simulink model "Clutch_control"  (R2020a)
settings: Solver=VariableStepAuto  StartTime=0.0  StopTime=10.0  RelTol=1e-3
undefined symbols (not defined in the file or in its folder): be, bv, Ie, Iv, lv, muk, mus, R
settings Model: Creator=DELL  LastModifiedBy=DELL

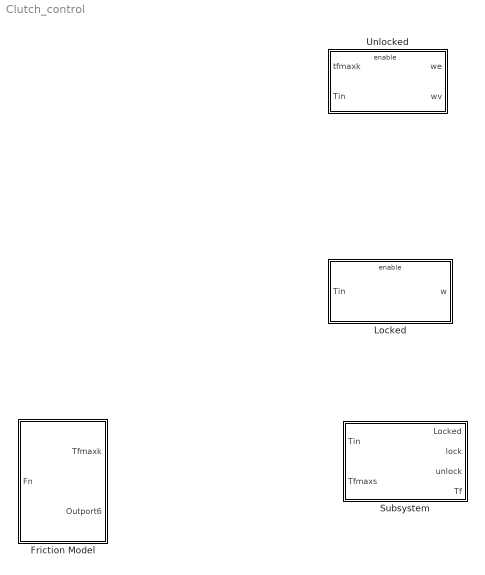
== system Clutch_control ==
  Friction Model : Subsystem
  Locked : Subsystem
  Subsystem : Subsystem
  Unlocked : Subsystem

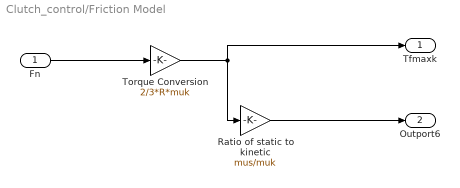
== system Clutch_control/Friction Model ==
  Fn : Inport
  Ratio of static to kinetic : Gain  Gain=mus/muk
  Torque Conversion : Gain  Gain=2/3*R*muk
  Tfmaxk : Outport
  Outport6 : Outport  Port=2
  wires:
  Torque Conversion/1 -> Tfmaxk/1, Ratio of static to kinetic/1
  Fn/1 -> Torque Conversion/1
  Ratio of static to kinetic/1 -> Outport6/1

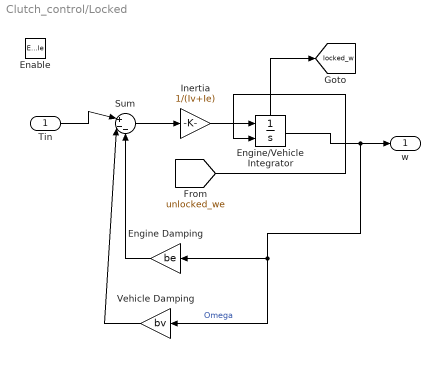
== system Clutch_control/Locked ==
  Tin : Inport
  Enable : EnablePort  StatesWhenEnabling=reset
  Engine Damping : Gain  Gain=be
  Engine/Vehicle Integrator : Integrator  InitialConditionSource=external  ShowStatePort=on
  Inertia : Gain  Gain=1/(Iv+Ie)
  Sum : Sum  Inputs=|+--
  Vehicle Damping : Gain  Gain=bv
  w : Outport
  tag scope: locked_w=global
  wires:
  Engine/Vehicle Integrator/1 -> w/1, Vehicle Damping/1, Engine Damping/1  "Omega"
  Inertia/1 -> Engine/Vehicle Integrator/1
  Engine/Vehicle Integrator/State -> [locked_w]
  [unlocked_we] -> Engine/Vehicle Integrator/2
  Engine Damping/1 -> Sum/3
  Tin/1 -> Sum/1
  Vehicle Damping/1 -> Sum/2
  Sum/1 -> Inertia/1

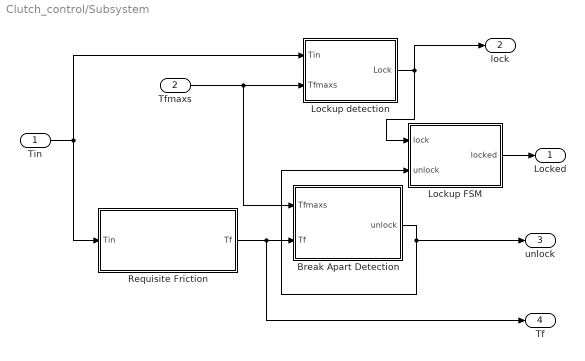
== system Clutch_control/Subsystem ==
  Tin : Inport
  Tfmaxs : Inport  Port=2
  Break Apart Detection : Subsystem
  Lockup FSM : Subsystem
  Lockup detection : Subsystem
  Requisite Friction : Subsystem
  Locked : Outport
  lock : Outport  Port=2
  unlock : Outport  Port=3
  Tf : Outport  Port=4
  wires:
  Tfmaxs/1 -> Break Apart Detection/1(Tfmaxs), Lockup detection/2(Tfmaxs)
  Tin/1 -> Lockup detection/1(Tin), Requisite Friction/1(Tin)
  Lockup detection/1(Lock) -> lock/1, Lockup FSM/1(lock)
  Requisite Friction/1(Tf) -> Tf/1, Break Apart Detection/2(Tf)
  Lockup FSM/1(locked) -> Locked/1
  Break Apart Detection/1(unlock) -> unlock/1, Lockup FSM/2(unlock)

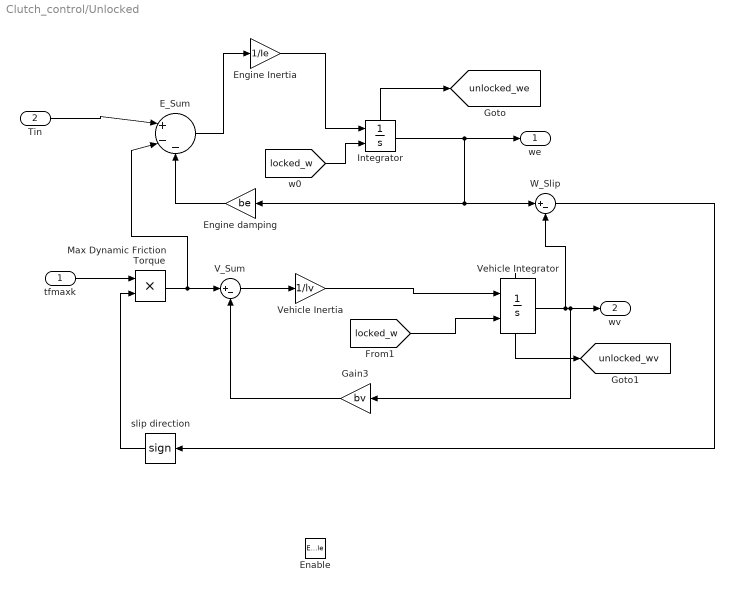
== system Clutch_control/Unlocked ==
  tfmaxk : Inport
  Tin : Inport  Port=2
  Enable : EnablePort  StatesWhenEnabling=reset  ShowOutputPort=on
  E_Sum : Sum  Inputs=|+--
  Engine Inertia : Gain  Gain=1/Ie
  Engine damping : Gain  Gain=be
  Gain3 : Gain  Gain=bv
  Integrator : Integrator  InitialConditionSource=external  ShowStatePort=on
  Max Dynamic Friction Torque : Product
  V_Sum : Sum  Inputs=|+-
  Vehicle Integrator : Integrator  InitialConditionSource=external  ShowStatePort=on
  Vehicle Inertia : Gain  Gain=1/lv
  W_Slip : Sum  Inputs=|+-
  slip direction : Signum
  we : Outport
  wv : Outport  Port=2
  tag scope: unlocked_we=global, unlocked_wv=global
  wires:
  W_Slip/1 -> slip direction/1
  Integrator/1 -> we/1, W_Slip/1, Engine damping/1
  Engine Inertia/1 -> Integrator/1
  tfmaxk/1 -> Max Dynamic Friction Torque/1
  Vehicle Integrator/State -> [unlocked_wv]
  slip direction/1 -> Max Dynamic Friction Torque/2
  Gain3/1 -> V_Sum/2
  Vehicle Integrator/1 -> W_Slip/2, wv/1, Gain3/1
  Tin/1 -> E_Sum/1
  V_Sum/1 -> Vehicle Inertia/1
  Integrator/State -> [unlocked_we]
  Max Dynamic Friction Torque/1 -> E_Sum/2, V_Sum/1
  [locked_w] -> Vehicle Integrator/2
  E_Sum/1 -> Engine Inertia/1
  Engine damping/1 -> E_Sum/3
  [locked_w] -> Integrator/2
  Vehicle Inertia/1 -> Vehicle Integrator/1

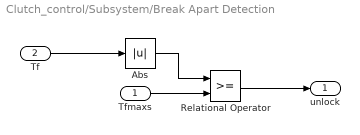
== system Clutch_control/Subsystem/Break Apart Detection ==
  Tfmaxs : Inport
  Tf : Inport  Port=2
  Abs : Abs
  Relational Operator : RelationalOperator  OutDataTypeStr=boolean  RndMeth=Simplest
  unlock : Outport
  wires:
  Abs/1 -> Relational Operator/1
  Tf/1 -> Abs/1
  Relational Operator/1 -> unlock/1
  Tfmaxs/1 -> Relational Operator/2

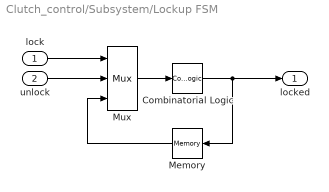
== system Clutch_control/Subsystem/Lockup FSM ==
  lock : Inport
  unlock : Inport  Port=2
  Combinatorial Logic : CombinatorialLogic  TruthTable=[0;1;0;0;1;1;1;0]
  Memory : Memory
  Mux : Mux  Inputs=3
  locked : Outport  InitialOutput=0  VectorParamsAs1DForOutWhenUnconnected=off
  wires:
  Memory/1 -> Mux/3
  unlock/1 -> Mux/2
  Combinatorial Logic/1 -> locked/1, Memory/1
  lock/1 -> Mux/1
  Mux/1 -> Combinatorial Logic/1

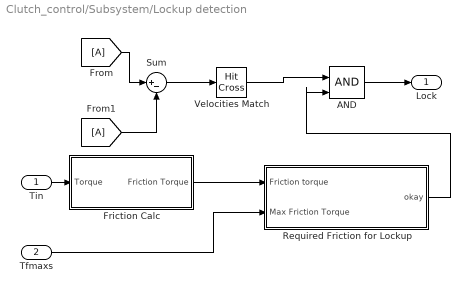
== system Clutch_control/Subsystem/Lockup detection ==
  Tin : Inport
  Tfmaxs : Inport  Port=2
  " Velocities Match" : HitCross
  AND : Logic  IconShape=distinctive  AllPortsSameDT=off  OutDataTypeStr=boolean
  Friction Calc : Subsystem
  Required Friction for Lockup : Subsystem
  Sum : Sum  Inputs=|+-
  Lock : Outport
  wires:
  Sum/1 -> " Velocities Match"/1
  Required Friction for Lockup/1(okay) -> AND/2
  Tin/1 -> Friction Calc/1(Torque)
  Friction Calc/1(Friction Torque) -> Required Friction for Lockup/1(Friction torque)
  AND/1 -> Lock/1
  Tfmaxs/1 -> Required Friction for Lockup/2(Max Friction Torque)
  [A] -> Sum/2
  [A] -> Sum/1
  " Velocities Match"/1 -> AND/1

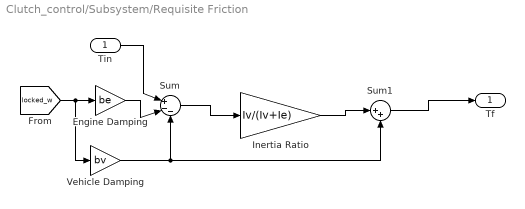
== system Clutch_control/Subsystem/Requisite Friction ==
  Tin : Inport
  Engine Damping : Gain  Gain=be
  Inertia Ratio : Gain  Gain=Iv/(Iv+Ie)
  Sum : Sum  Inputs=|+--
  Sum1 : Sum  Inputs=|++
  Vehicle Damping : Gain  Gain=bv
  Tf : Outport
  wires:
  Sum1/1 -> Tf/1
  [locked_w] -> Vehicle Damping/1, Engine Damping/1
  Inertia Ratio/1 -> Sum1/1
  Vehicle Damping/1 -> Sum1/2, Sum/3
  Sum/1 -> Inertia Ratio/1
  Engine Damping/1 -> Sum/2
  Tin/1 -> Sum/1

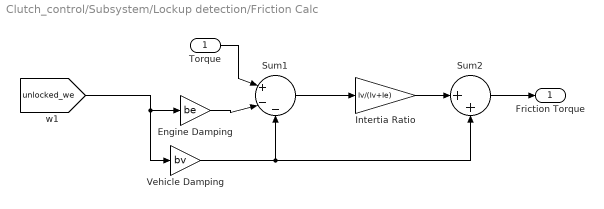
== system Clutch_control/Subsystem/Lockup detection/Friction Calc ==
  Torque : Inport
  Engine Damping : Gain  Gain=be
  Intertia Ratio : Gain  Gain=Iv/(Iv+Ie)
  Sum1 : Sum  Inputs=|+--
  Sum2 : Sum  Inputs=|++
  Vehicle Damping : Gain  Gain=bv
  Friction Torque : Outport
  wires:
  [unlocked_we] -> Vehicle Damping/1, Engine Damping/1
  Engine Damping/1 -> Sum1/2
  Intertia Ratio/1 -> Sum2/1
  Sum2/1 -> Friction Torque/1
  Vehicle Damping/1 -> Sum2/2, Sum1/3
  Sum1/1 -> Intertia Ratio/1
  Torque/1 -> Sum1/1

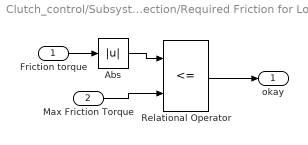
== system Clutch_control/Subsystem/Lockup detection/Required Friction for Lockup ==
  Friction torque : Inport
  Max Friction Torque : Inport  Port=2
  Abs : Abs
  Relational Operator : RelationalOperator  Operator=<=  OutDataTypeStr=boolean  RndMeth=Simplest
  okay : Outport
  wires:
  Relational Operator/1 -> okay/1
  Max Friction Torque/1 -> Relational Operator/2
  Abs/1 -> Relational Operator/1
  Friction torque/1 -> Abs/1
